simulink model "PMSM_PI_selfmode"  (R2023a)
settings: Solver=ode23tb  StartTime=0.0  StopTime=0.5  FixedStep=Ts  RelTol=1e-3  EnableMultiTasking=on
InitFcn:
  | Ts = 1e-6;
libraries: powerlib_extras x3, spsVoltageMeasurementLib x3, spsGroundLib x2, spsDCVoltageSourceLib x1, spsUniversalBridgeLib x1, simulink x1, spspowerguiLib x1
settings Model: Creator=Administrator  LastModifiedBy=Guoguo
settings SolverCC: AlgebraicLoopSolver=TrustRegion
settings DataIOCC: LimitDataPoints=on  SaveFormat=Array  SignalLoggingSaveFormat=ModelDataLogs  ReturnWorkspaceOutputs=off
settings OptimizationCC: ExpressionDepthLimit=2147483647  InitFltsAndDblsToZero=on  LifeSpan=inf
settings DebuggingCC: SaveWithParameterizedLinksMsg=none  UnderspecifiedInitializationDetection=Classic  MergeDetectMultiDrivingBlocksExec=none  SolverPrmCheckMsg=warning  FcnCallInpInsideContextMsg=warning  UnconnectedInputMsg=warning  UnconnectedOutputMsg=warning  UnconnectedLineMsg=warning  StateNameClashWarn=warning  SFUnexpectedBacktrackingDiag=warning  SFNoUnconditionalDefaultTransitionDiag=warning  SFExecutionAtInitializationDiag=none  ArithmeticOperatorsInVariantConditions=warning
settings HardwareCC: ProdBitPerPointer=32  ProdBitPerSizeT=32  ProdBitPerPtrDiffT=32  ProdLargestAtomicFloat=None  ProdIntDivRoundTo=Undefined  ProdEndianess=Unspecified  ProdWordSize=32  ProdHWDeviceType=32-bit Generic
settings ModelReferenceCC: EnableRefExpFcnMdlSchedulingChecks=on  PropagateSignalLabelsOutOfModel=off
settings SFSimCC: SimUseLocalCustomCode=off  CustomCodeUndefinedFunction=UseInterfaceOnly
settings RTWCC: RTWUseLocalCustomCode=off
settings CodeAppCC: StateflowObjectComments=on
settings GRTTargetCC: TargetFcnLib=ansi_tfl_tmw.mat  TargetLangStandard=C89/C90 (ANSI)  CombineOutputUpdateFcns=off  GRTInterface=on
settings ConfigComp: CovMetricSettings=dw  CovSaveCumulativeToWorkspaceVar=on  CovSaveSingleToWorkspaceVar=on  CovExternalEMLEnable=off  CovSFcnEnable=off
settings SimscapeCC: SimscapeNormalizeSystem=off

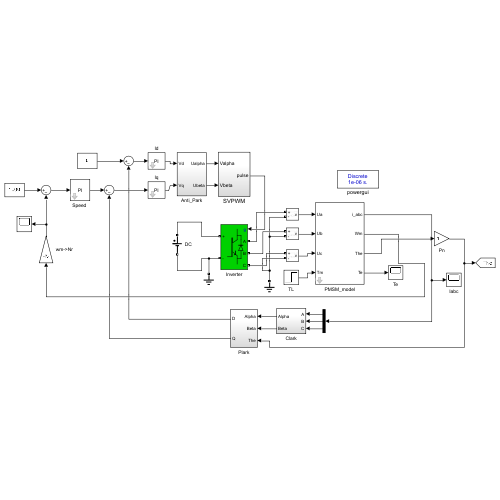
[thumbnail: Simulink's stored preview of the top-level diagram]
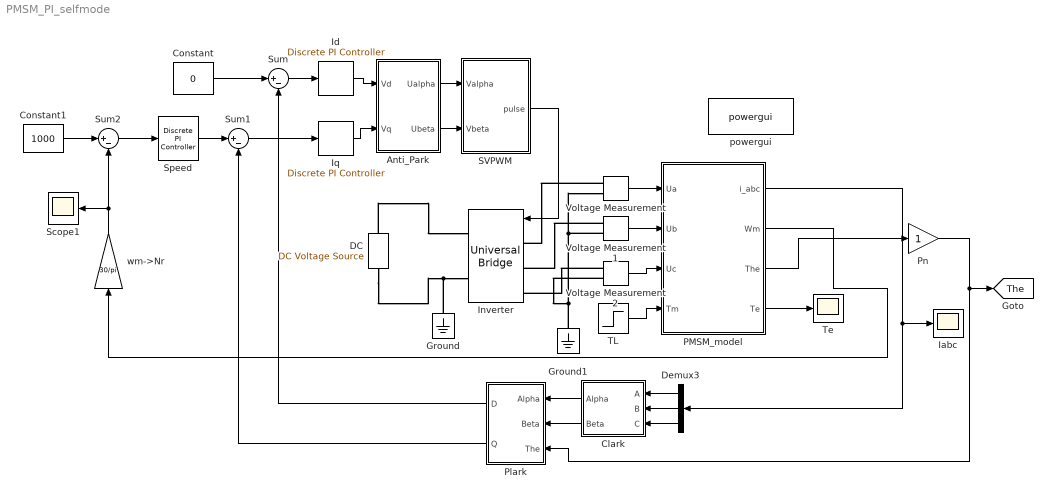
== system PMSM_PI_selfmode ==
  Anti_Park : Subsystem
  Clark : Subsystem
  Constant : Constant  Value=0
  Constant1 : Constant  Value=1000
  "DC " : spsDCVoltageSourceLib/DC Voltage Source  Amplitude=350  Measurements=None
  Demux3 : Demux  Outputs=3
  Ground : spsGroundLib/Ground  LConnTagsString=a
  Ground1 : spsGroundLib/Ground  LConnTagsString=a
  Iabc : Scope
  Id : powerlib_extras/Discrete  Control Blocks/Discrete PI Controller  Kp=8.8e-3*2200  Ki=2.875*2200  Par_Limits=[200 -200]  Init=0  Ts=Ts
  Inverter : spsUniversalBridgeLib/Universal Bridge  Arms=3  SnubberResistance=1e5  SnubberCapacitance=inf  Device=IGBT / Diodes  Ron=1e-3  Lon=0  ForwardVoltages="[  0  0  ]"  ForwardVoltage=0  GTOparameters=[ 10e-6 , 20e-6 ]  IGBTparameters=[ 1e-6 , 2e-6 ]  Measurements=None  Measurements_2=None  converterType=Rectifier
  Iq : powerlib_extras/Discrete  Control Blocks/Discrete PI Controller  Kp=8.5e-3*2200  Ki=2.875*20000  Par_Limits=[200 -200]  Init=0  Ts=Ts
  PMSM_model : Subsystem  mask{Ld=8.5e-3, Lq=8.5e-3, R=2.875, Pn=2, flux=0.533, B=0.0001, J=0.008}
      mask prompts: Ld "d-Inductances(Ld)"; Lq "q-Inductances(Lq)"; R "resistance(R)"; Pn "pole pairs(Pn)"; flux "Flux linkage(flux)"; B "viscous damping(B)"; J "Inertia(J)"
  Plark : Subsystem
  Pn : Gain
  SVPWM : Subsystem
  Scope1 : Scope
  "Speed " : powerlib_extras/Discrete  Control Blocks/Discrete PI Controller  Kp=0.2  Ki=10/4  Par_Limits=[15 -15]  Init=0  Ts=Ts
  Sum : Sum  Inputs=|+-
  Sum1 : Sum  Inputs=|+-
  Sum2 : Sum  Inputs=|+-
  TL : Step  Time=0.3  After=5  SampleTime=0
  Te : Scope
  Voltage Measurement : spsVoltageMeasurementLib/Voltage Measurement  PhasorSimulation=off  OutputType=Complex  PSBequivalent=0
  Voltage Measurement1 : spsVoltageMeasurementLib/Voltage Measurement  PhasorSimulation=off  OutputType=Complex  PSBequivalent=0
  Voltage Measurement2 : spsVoltageMeasurementLib/Voltage Measurement  PhasorSimulation=off  OutputType=Complex  PSBequivalent=0
  powergui : spspowerguiLib/powergui  SimulationMode=Discrete  SampleTime=Ts  frequency=60  Iterations=50  frequencyindice=0  Pbase=100e6  ErrMax=1e-4  UnitsV=kV  UnitsW=MW  buscounter=0  FunctionMessages=off  echomessages=off  EnableUseOfTLC=off  CurrentSourceSwitches=off  DisableSnubberDevices=off  DisableRonSwitches=off  DisableVfSwitches=off  DisplayEquations=off  AutomaticDiscreteSolvers=off  SolverType=Tustin/Backward Euler (TBE)  Interpol=off  ExternalGateDelay=off  methode=off  Ts=0  x0status=blocks  SPID=off  SwTol=0  HookPort=off  NonlinearTolerance=1e-4  nMaxIteration=100  ContinueOnMaxIteration=off  RestoreLinks=warning  ResistiveCurrentMeasurement=off  Frange=[0:2:500]  Ylog=off  Xlog=on  ShowGrid=off  save=off  variable=ZData  structure=0  ZoomFFT=off  StartTime=0.0  cycles=1  DisplayStyle=1  fundamental=60  FreqAxis=off  MaxFrequency=1000  frequencyindicesteady=1  RmsSteady=1  display=off
  wm->Nr : Gain  Gain=30/pi
  tag scope: The=global
  wires:
  SVPWM/1(pulse) -> Inverter/1
  Id/1 -> Anti_Park/1(Vd)
  Iq/1 -> Anti_Park/2(Vq)
  Sum/1 -> Id/1
  Sum1/1 -> Iq/1
  Sum2/1 -> "Speed "/1
  Constant1/1 -> Sum2/1
  "Speed "/1 -> Sum1/1
  wm->Nr/1 -> Sum2/2, Scope1/1
  Anti_Park/1(Ualpha) -> SVPWM/1(Valpha)
  Anti_Park/2(Ubeta) -> SVPWM/2(Vbeta)
  Constant/1 -> Sum/1
  Pn/1 -> Plark/3(The), [The]
  PMSM_model/3(The) -> Pn/1
  PMSM_model/2(Wm) -> wm->Nr/1
  PMSM_model/1(i_abc) -> Iabc/1, Demux3/1
  Clark/2(Beta) -> Plark/2(Beta)
  Clark/1(Alpha) -> Plark/1(Alpha)
  Demux3/1 -> Clark/1(A)
  Demux3/2 -> Clark/2(B)
  Demux3/3 -> Clark/3(C)
  Plark/1(D) -> Sum/2
  Plark/2(Q) -> Sum1/2
  Voltage Measurement/1 -> PMSM_model/1(Ua)
  Voltage Measurement1/1 -> PMSM_model/2(Ub)
  Voltage Measurement2/1 -> PMSM_model/3(Uc)
  TL/1 -> PMSM_model/4(Tm)
  PMSM_model/4(Te) -> Te/1
  connections:
  "DC "/RConn1 -- Inverter/RConn1
  "DC "/LConn1 -- Ground/LConn1 -- Inverter/RConn2
  Voltage Measurement/LConn1 -- Inverter/LConn1
  Voltage Measurement1/LConn1 -- Inverter/LConn2
  Voltage Measurement2/LConn1 -- Inverter/LConn3
  Ground1/LConn1 -- Voltage Measurement2/LConn2 -- Voltage Measurement1/LConn2 -- Voltage Measurement/LConn2

== system PMSM_PI_selfmode/Anti_Park ==
  Vd : Inport
  Vq : Inport  Port=2
  Fcn : Fcn  Expr=cos(u[1])*u[2]-sin(u[1])*u[3]
  Fcn1 : Fcn  Expr=sin(u[1])*u[2]+cos(u[1])*u[3]
  Mux1 : Mux  Inputs=3
  Ualpha : Outport  VectorParamsAs1DForOutWhenUnconnected=off
  Ubeta : Outport  Port=2  VectorParamsAs1DForOutWhenUnconnected=off
  wires:
  Fcn1/1 -> Ubeta/1
  Fcn/1 -> Ualpha/1
  Mux1/1 -> Fcn/1, Fcn1/1
  Vd/1 -> Mux1/2
  Vq/1 -> Mux1/3
  [The] -> Mux1/1

== system PMSM_PI_selfmode/Clark ==
  A : Inport
  B : Inport  Port=2
  C : Inport  Port=3
  Mux : Mux  Inputs=3
  alpha : Fcn  Expr=(u(1)-0.5*(u(2)+u(3)))*2/3
  beta : Fcn  Expr=sqrt(3)/2*(u(2)-u(3))*2/3
  Alpha : Outport  VectorParamsAs1DForOutWhenUnconnected=off
  Beta : Outport  Port=2  VectorParamsAs1DForOutWhenUnconnected=off
  wires:
  alpha/1 -> Alpha/1
  B/1 -> Mux/2
  C/1 -> Mux/3
  A/1 -> Mux/1
  Mux/1 -> beta/1, alpha/1
  beta/1 -> Beta/1

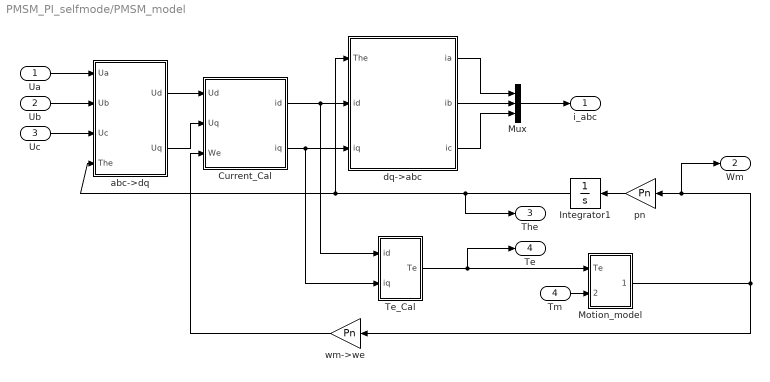
== system PMSM_PI_selfmode/PMSM_model ==
  Ua : Inport
  Ub : Inport  Port=2
  Uc : Inport  Port=3
  Tm : Inport  Port=4
  Current_Cal : Subsystem
  Integrator1 : Integrator
  Motion_model : Subsystem
  Mux : Mux  Inputs=3
  Te_Cal : Subsystem
  abc->dq : Subsystem
  dq->abc : Subsystem
  pn : Gain  Gain=Pn  SaturateOnIntegerOverflow=on  OutDataTypeStr=Inherit: Same as input  ParamDataTypeStr=Inherit: Same as input
  wm->we : Gain  Gain=Pn  SaturateOnIntegerOverflow=on  OutDataTypeStr=Inherit: Same as input  ParamDataTypeStr=Inherit: Same as input
  i_abc : Outport  VectorParamsAs1DForOutWhenUnconnected=off
  Wm : Outport  Port=2  VectorParamsAs1DForOutWhenUnconnected=off
  The : Outport  Port=3  VectorParamsAs1DForOutWhenUnconnected=off
  Te : Outport  Port=4  VectorParamsAs1DForOutWhenUnconnected=off
  wires:
  Ua/1 -> abc->dq/1(Ua)
  abc->dq/1(Ud) -> Current_Cal/1(Ud)
  abc->dq/2(Uq) -> Current_Cal/2(Uq)
  Current_Cal/1(id) -> Te_Cal/1(id), dq->abc/2(id)
  Current_Cal/2(iq) -> Te_Cal/2(iq), dq->abc/3(iq)
  Integrator1/1 -> abc->dq/4(The), dq->abc/1(The), The/1
  dq->abc/1(ia) -> Mux/1
  pn/1 -> Integrator1/1
  Uc/1 -> abc->dq/3(Uc)
  Ub/1 -> abc->dq/2(Ub)
  dq->abc/3(ic) -> Mux/3
  Mux/1 -> i_abc/1
  dq->abc/2(ib) -> Mux/2
  wm->we/1 -> Current_Cal/3(We)
  Motion_model/1(wm) -> wm->we/1, Wm/1, pn/1
  Te_Cal/1(Te) -> Te/1, Motion_model/1(Te)
  Tm/1 -> Motion_model/2(Tm)

== system PMSM_PI_selfmode/Plark ==
  Alpha : Inport
  Beta : Inport  Port=2
  The : Inport  Port=3
  Mux : Mux  Inputs=3
  d : Fcn  Expr=u(1)*cos(u(3))+u(2)*sin(u(3))
  q : Fcn  Expr=-u(1)*sin(u(3))+u(2)*cos(u(3))
  D : Outport  VectorParamsAs1DForOutWhenUnconnected=off
  Q : Outport  Port=2  VectorParamsAs1DForOutWhenUnconnected=off
  wires:
  d/1 -> D/1
  Beta/1 -> Mux/2
  The/1 -> Mux/3
  Alpha/1 -> Mux/1
  Mux/1 -> q/1, d/1
  q/1 -> Q/1

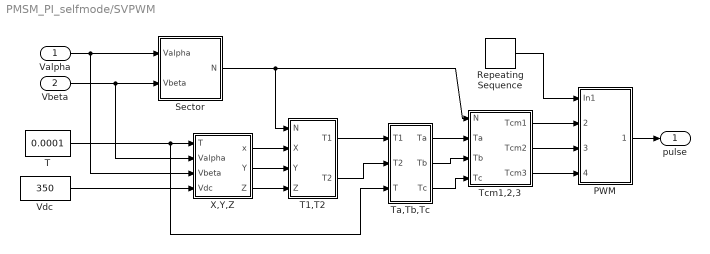
== system PMSM_PI_selfmode/SVPWM ==
  Valpha : Inport
  Vbeta : Inport  Port=2
  PWM : Subsystem
  Repeating Sequence : simulink/Sources/Repeating Sequence  rep_seq_t=[0 0.00005 0.0001]  rep_seq_y=[0 0.00005 0]
  Sector : Subsystem
  T : Constant  Value=0.0001
  T1,T2 : Subsystem
  Ta,Tb,Tc : Subsystem
  Tcm1,2,3 : Subsystem
  Vdc : Constant  Value=350
  X,Y,Z : Subsystem
  pulse : Outport  VectorParamsAs1DForOutWhenUnconnected=off
  wires:
  PWM/1(PWM) -> pulse/1
  Repeating Sequence/1 -> PWM/1(In1)
  Tcm1,2,3/3(Tcm3) -> PWM/4(Tcm3)
  Tcm1,2,3/2(Tcm2) -> PWM/3(Tcm2)
  Tcm1,2,3/1(Tcm1) -> PWM/2(Tcm1)
  Ta,Tb,Tc/3(Tc) -> Tcm1,2,3/4(Tc)
  Ta,Tb,Tc/2(Tb) -> Tcm1,2,3/3(Tb)
  Ta,Tb,Tc/1(Ta) -> Tcm1,2,3/2(Ta)
  T1,T2/2(T2) -> Ta,Tb,Tc/2(T2)
  T1,T2/1(T1) -> Ta,Tb,Tc/1(T1)
  X,Y,Z/3(Z) -> T1,T2/4(Z)
  X,Y,Z/2(Y) -> T1,T2/3(Y)
  X,Y,Z/1(x) -> T1,T2/2(X)
  Sector/1(N) -> T1,T2/1(N), Tcm1,2,3/1(N)
  Vdc/1 -> X,Y,Z/4(Vdc)
  T/1 -> Ta,Tb,Tc/3(T), X,Y,Z/1(T)
  Vbeta/1 -> X,Y,Z/2(Valpha), Sector/2(Vbeta)
  Valpha/1 -> X,Y,Z/3(Vbeta), Sector/1(Valpha)

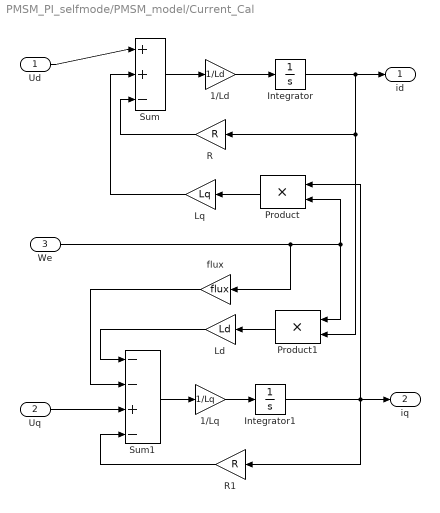
== system PMSM_PI_selfmode/PMSM_model/Current_Cal ==
  Ud : Inport
  Uq : Inport  Port=2
  We : Inport  Port=3
  1/Ld : Gain  Gain=1/Ld  SaturateOnIntegerOverflow=on  OutDataTypeStr=Inherit: Same as input  ParamDataTypeStr=Inherit: Same as input
  1/Lq : Gain  Gain=1/Lq  SaturateOnIntegerOverflow=on  OutDataTypeStr=Inherit: Same as input  ParamDataTypeStr=Inherit: Same as input
  Integrator : Integrator  InitialCondition=0.01
  Integrator1 : Integrator
  Ld : Gain  Gain=Ld  SaturateOnIntegerOverflow=on  OutDataTypeStr=Inherit: Same as input  ParamDataTypeStr=Inherit: Same as input
  Lq : Gain  Gain=Lq  SaturateOnIntegerOverflow=on  OutDataTypeStr=Inherit: Same as input  ParamDataTypeStr=Inherit: Same as input
  Product : Product  SaturateOnIntegerOverflow=on  OutDataTypeStr=Inherit: Same as first input
  Product1 : Product  SaturateOnIntegerOverflow=on  OutDataTypeStr=Inherit: Same as first input
  R : Gain  Gain=R  SaturateOnIntegerOverflow=on  OutDataTypeStr=Inherit: Same as input  ParamDataTypeStr=Inherit: Same as input
  R1 : Gain  Gain=R  SaturateOnIntegerOverflow=on  OutDataTypeStr=Inherit: Same as input  ParamDataTypeStr=Inherit: Same as input
  Sum : Sum  Inputs=|++-  SaturateOnIntegerOverflow=on
  Sum1 : Sum  Inputs=--+-  SaturateOnIntegerOverflow=on
  flux : Gain  Gain=flux  SaturateOnIntegerOverflow=on  OutDataTypeStr=Inherit: Same as input  ParamDataTypeStr=Inherit: Same as input
  id : Outport  VectorParamsAs1DForOutWhenUnconnected=off
  iq : Outport  Port=2  VectorParamsAs1DForOutWhenUnconnected=off
  wires:
  Ud/1 -> Sum/1
  Sum/1 -> 1/Ld/1
  1/Ld/1 -> Integrator/1
  Integrator/1 -> Product1/2, R/1, id/1
  Product/1 -> Lq/1
  Lq/1 -> Sum/2
  We/1 -> Product/2, Product1/1, flux/1
  R/1 -> Sum/3
  R1/1 -> Sum1/4
  1/Lq/1 -> Integrator1/1
  Sum1/1 -> 1/Lq/1
  Integrator1/1 -> R1/1, Product/1, iq/1
  Product1/1 -> Ld/1
  Ld/1 -> Sum1/1
  Uq/1 -> Sum1/3
  flux/1 -> Sum1/2

== system PMSM_PI_selfmode/PMSM_model/Motion_model ==
  Te : Inport
  Tm : Inport  Port=2
  1/J : Gain  Gain=1/J  SaturateOnIntegerOverflow=on  OutDataTypeStr=Inherit: Same as input  ParamDataTypeStr=Inherit: Same as input
  B : Gain  Gain=B  SaturateOnIntegerOverflow=on  OutDataTypeStr=Inherit: Same as input  ParamDataTypeStr=Inherit: Same as input
  Integrator : Integrator
  Memory : Memory
  Sum1 : Sum  Inputs=|+--  SaturateOnIntegerOverflow=on
  wm : Outport  VectorParamsAs1DForOutWhenUnconnected=off
  wires:
  Tm/1 -> Sum1/3
  Sum1/1 -> 1/J/1
  B/1 -> Sum1/2
  1/J/1 -> Integrator/1
  Te/1 -> Sum1/1
  Integrator/1 -> Memory/1, wm/1
  Memory/1 -> B/1

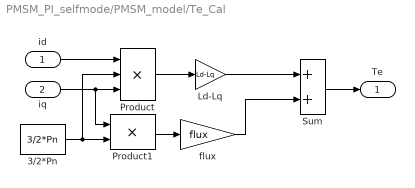
== system PMSM_PI_selfmode/PMSM_model/Te_Cal ==
  id : Inport
  iq : Inport  Port=2
  3/2*Pn : Constant  Value=3/2*Pn
  Ld-Lq : Gain  Gain=Ld-Lq  SaturateOnIntegerOverflow=on  OutDataTypeStr=Inherit: Same as input  ParamDataTypeStr=Inherit: Same as input
  Product : Product  Inputs=3  SaturateOnIntegerOverflow=on  OutDataTypeStr=Inherit: Same as first input
  Product1 : Product  SaturateOnIntegerOverflow=on  OutDataTypeStr=Inherit: Same as first input
  Sum : Sum  SaturateOnIntegerOverflow=on
  flux : Gain  Gain=flux  SaturateOnIntegerOverflow=on  OutDataTypeStr=Inherit: Same as input  ParamDataTypeStr=Inherit: Same as input
  Te : Outport  VectorParamsAs1DForOutWhenUnconnected=off
  wires:
  iq/1 -> Product1/1, Product/3
  id/1 -> Product/1
  Ld-Lq/1 -> Sum/1
  Product/1 -> Ld-Lq/1
  flux/1 -> Sum/2
  Product1/1 -> flux/1
  Sum/1 -> Te/1
  3/2*Pn/1 -> Product/2, Product1/2

== system PMSM_PI_selfmode/PMSM_model/abc->dq ==
  Ua : Inport
  Ub : Inport  Port=2
  Uc : Inport  Port=3
  The : Inport  Port=4
  Mux : Mux
  d : Fcn  Expr=(u(1)*cos(u(4))+u(2)*cos(u(4)-2/3*pi)+u(3)*cos(u(4)+2/3*pi))*2/3
  q : Fcn  Expr=-(u(1)*sin(u(4))+u(2)*sin(u(4)-2/3*pi)+u(3)*sin(u(4)+2/3*pi))*2/3
  Ud : Outport  VectorParamsAs1DForOutWhenUnconnected=off
  Uq : Outport  Port=2  VectorParamsAs1DForOutWhenUnconnected=off
  wires:
  Mux/1 -> q/1, d/1
  Ua/1 -> Mux/1
  Ub/1 -> Mux/2
  d/1 -> Ud/1
  The/1 -> Mux/4
  Uc/1 -> Mux/3
  q/1 -> Uq/1

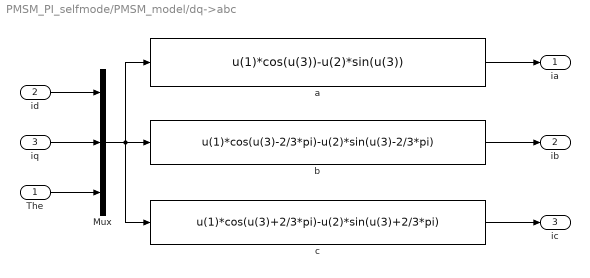
== system PMSM_PI_selfmode/PMSM_model/dq->abc ==
  The : Inport
  id : Inport  Port=2
  iq : Inport  Port=3
  Mux : Mux  Inputs=3
  a : Fcn  Expr=u(1)*cos(u(3))-u(2)*sin(u(3))
  b : Fcn  Expr=u(1)*cos(u(3)-2/3*pi)-u(2)*sin(u(3)-2/3*pi)
  c : Fcn  Expr=u(1)*cos(u(3)+2/3*pi)-u(2)*sin(u(3)+2/3*pi)
  ia : Outport  VectorParamsAs1DForOutWhenUnconnected=off
  ib : Outport  Port=2  VectorParamsAs1DForOutWhenUnconnected=off
  ic : Outport  Port=3  VectorParamsAs1DForOutWhenUnconnected=off
  wires:
  b/1 -> ib/1
  The/1 -> Mux/3
  a/1 -> ia/1
  id/1 -> Mux/1
  iq/1 -> Mux/2
  Mux/1 -> c/1, a/1, b/1
  c/1 -> ic/1

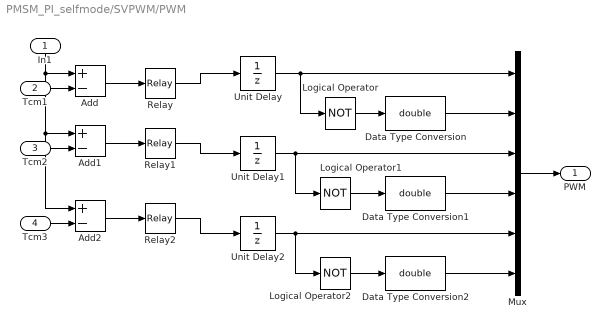
== system PMSM_PI_selfmode/SVPWM/PWM ==
  In1 : Inport
  Tcm1 : Inport  Port=2
  Tcm2 : Inport  Port=3
  Tcm3 : Inport  Port=4
  Add : Sum  Inputs=+-
  Add1 : Sum  Inputs=+-
  Add2 : Sum  Inputs=+-
  Data Type Conversion : DataTypeConversion  OutDataTypeStr=double  SaturateOnIntegerOverflow=off  RndMeth=Floor
  Data Type Conversion1 : DataTypeConversion  OutDataTypeStr=double  SaturateOnIntegerOverflow=off  RndMeth=Floor
  Data Type Conversion2 : DataTypeConversion  OutDataTypeStr=double  SaturateOnIntegerOverflow=off  RndMeth=Floor
  Logical Operator : Logic  Operator=NOT  AllPortsSameDT=off  OutDataTypeStr=boolean
  Logical Operator1 : Logic  Operator=NOT  AllPortsSameDT=off  OutDataTypeStr=boolean
  Logical Operator2 : Logic  Operator=NOT  AllPortsSameDT=off  OutDataTypeStr=boolean
  Mux : Mux  Inputs=6
  Relay : Relay  OffSwitchValue=-eps
  Relay1 : Relay  OffSwitchValue=-eps
  Relay2 : Relay  OffSwitchValue=-eps
  Unit Delay : UnitDelay  SampleTime=-1  HasFrameUpgradeWarning=on
  Unit Delay1 : UnitDelay  SampleTime=-1  HasFrameUpgradeWarning=on
  Unit Delay2 : UnitDelay  SampleTime=-1  HasFrameUpgradeWarning=on
  PWM : Outport  VectorParamsAs1DForOutWhenUnconnected=off
  wires:
  Tcm3/1 -> Add2/2
  Tcm2/1 -> Add1/2
  Tcm1/1 -> Add/2
  Relay2/1 -> Unit Delay2/1
  Relay1/1 -> Unit Delay1/1
  Relay/1 -> Unit Delay/1
  Unit Delay2/1 -> Mux/5, Logical Operator2/1
  Unit Delay1/1 -> Mux/3, Logical Operator1/1
  Unit Delay/1 -> Logical Operator/1, Mux/1
  Mux/1 -> PWM/1
  Data Type Conversion/1 -> Mux/2
  Data Type Conversion1/1 -> Mux/4
  Data Type Conversion2/1 -> Mux/6
  Logical Operator2/1 -> Data Type Conversion2/1
  Logical Operator1/1 -> Data Type Conversion1/1
  Logical Operator/1 -> Data Type Conversion/1
  Add1/1 -> Relay1/1
  Add2/1 -> Relay2/1
  Add/1 -> Relay/1
  In1/1 -> Add/1, Add2/1, Add1/1

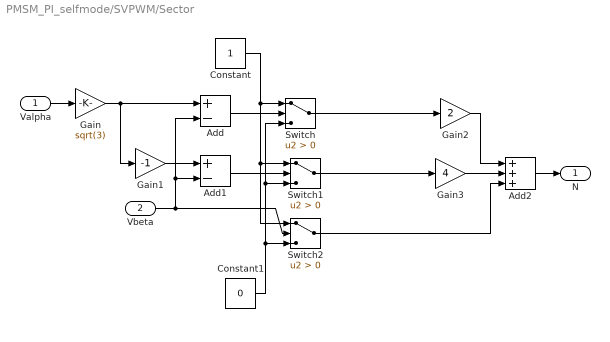
== system PMSM_PI_selfmode/SVPWM/Sector ==
  Valpha : Inport
  Vbeta : Inport  Port=2
  Add : Sum  Inputs=+-
  Add1 : Sum  Inputs=+-
  Add2 : Sum  Inputs=+++
  Constant : Constant
  Constant1 : Constant  Value=0
  Gain : Gain  Gain=sqrt(3)
  Gain1 : Gain  Gain=-1
  Gain2 : Gain  Gain=2
  Gain3 : Gain  Gain=4
  Switch : Switch  Criteria=u2 > Threshold  SaturateOnIntegerOverflow=off  InputSameDT=off
  Switch1 : Switch  Criteria=u2 > Threshold  SaturateOnIntegerOverflow=off  InputSameDT=off
  Switch2 : Switch  Criteria=u2 > Threshold  SaturateOnIntegerOverflow=off  InputSameDT=off
  N : Outport  VectorParamsAs1DForOutWhenUnconnected=off
  wires:
  Add2/1 -> N/1
  Valpha/1 -> Gain/1
  Gain3/1 -> Add2/2
  Gain2/1 -> Add2/1
  Add1/1 -> Switch1/2
  Gain1/1 -> Add1/1
  Switch1/1 -> Gain3/1
  Switch2/1 -> Add2/3
  Switch/1 -> Gain2/1
  Add/1 -> Switch/2
  Gain/1 -> Gain1/1, Add/1
  Constant1/1 -> Switch/3, Switch1/3, Switch2/3
  Constant/1 -> Switch1/1, Switch2/1, Switch/1
  Vbeta/1 -> Add1/2, Add/2, Switch2/2

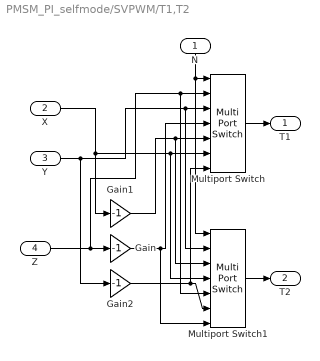
== system PMSM_PI_selfmode/SVPWM/T1,T2 ==
  N : Inport
  X : Inport  Port=2
  Y : Inport  Port=3
  Z : Inport  Port=4
  Gain : Gain  Gain=-1
  Gain1 : Gain  Gain=-1
  Gain2 : Gain  Gain=-1
  Multiport Switch : MultiPortSwitch  Inputs=6  SaturateOnIntegerOverflow=off  InputSameDT=off
  Multiport Switch1 : MultiPortSwitch  Inputs=6  SaturateOnIntegerOverflow=off  InputSameDT=off
  T1 : Outport  VectorParamsAs1DForOutWhenUnconnected=off
  T2 : Outport  Port=2  VectorParamsAs1DForOutWhenUnconnected=off
  wires:
  Multiport Switch1/1 -> T2/1
  Multiport Switch/1 -> T1/1
  Gain2/1 -> Multiport Switch/7, Multiport Switch1/6
  Gain1/1 -> Multiport Switch1/3, Multiport Switch/5
  X/1 -> Gain1/1, Multiport Switch/6, Multiport Switch1/4
  Gain/1 -> Multiport Switch1/7, Multiport Switch/4
  Y/1 -> Gain2/1, Multiport Switch1/2, Multiport Switch/3
  Z/1 -> Multiport Switch/2, Multiport Switch1/5, Gain/1
  N/1 -> Multiport Switch/1, Multiport Switch1/1

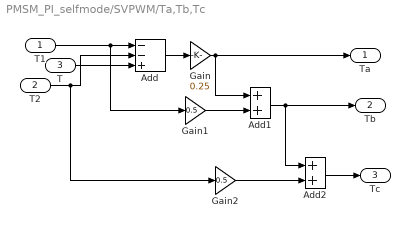
== system PMSM_PI_selfmode/SVPWM/Ta,Tb,Tc ==
  T1 : Inport
  T2 : Inport  Port=2
  T : Inport  Port=3
  Add : Sum  Inputs=--+
  Add1 : Sum
  Add2 : Sum
  Gain : Gain  Gain=0.25
  Gain1 : Gain  Gain=0.5
  Gain2 : Gain  Gain=0.5
  Ta : Outport  VectorParamsAs1DForOutWhenUnconnected=off
  Tb : Outport  Port=2  VectorParamsAs1DForOutWhenUnconnected=off
  Tc : Outport  Port=3  VectorParamsAs1DForOutWhenUnconnected=off
  wires:
  T/1 -> Add/3
  Add2/1 -> Tc/1
  Gain2/1 -> Add2/2
  Add1/1 -> Add2/1, Tb/1
  Gain1/1 -> Add1/2
  Gain/1 -> Add1/1, Ta/1
  Add/1 -> Gain/1
  T2/1 -> Add/2, Gain2/1
  T1/1 -> Add/1, Gain1/1

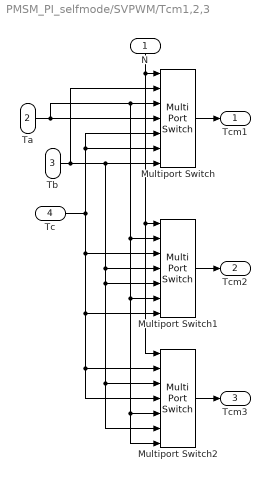
== system PMSM_PI_selfmode/SVPWM/Tcm1,2,3 ==
  N : Inport
  Ta : Inport  Port=2
  Tb : Inport  Port=3
  Tc : Inport  Port=4
  Multiport Switch : MultiPortSwitch  Inputs=6  SaturateOnIntegerOverflow=off  InputSameDT=off
  Multiport Switch1 : MultiPortSwitch  Inputs=6  SaturateOnIntegerOverflow=off  InputSameDT=off
  Multiport Switch2 : MultiPortSwitch  Inputs=6  SaturateOnIntegerOverflow=off  InputSameDT=off
  Tcm1 : Outport  VectorParamsAs1DForOutWhenUnconnected=off
  Tcm2 : Outport  Port=2  VectorParamsAs1DForOutWhenUnconnected=off
  Tcm3 : Outport  Port=3  VectorParamsAs1DForOutWhenUnconnected=off
  wires:
  Multiport Switch2/1 -> Tcm3/1
  Multiport Switch1/1 -> Tcm2/1
  Multiport Switch/1 -> Tcm1/1
  N/1 -> Multiport Switch2/1, Multiport Switch1/1, Multiport Switch/1
  Tc/1 -> Multiport Switch1/3, Multiport Switch1/7, Multiport Switch2/2, Multiport Switch2/4, Multiport Switch/5, Multiport Switch/6
  Ta/1 -> Multiport Switch/4, Multiport Switch/3, Multiport Switch1/2, Multiport Switch1/6, Multiport Switch2/5, Multiport Switch2/7
  Tb/1 -> Multiport Switch/2, Multiport Switch/7, Multiport Switch1/4, Multiport Switch1/5, Multiport Switch2/3, Multiport Switch2/6

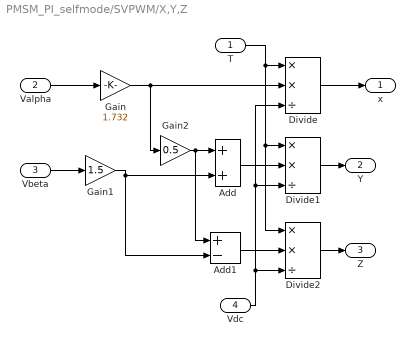
== system PMSM_PI_selfmode/SVPWM/X,Y,Z ==
  T : Inport
  Valpha : Inport  Port=2
  Vbeta : Inport  Port=3
  Vdc : Inport  Port=4
  Add : Sum
  Add1 : Sum  Inputs=+-
  Divide : Product  Inputs=**/
  Divide1 : Product  Inputs=**/
  Divide2 : Product  Inputs=**/
  Gain : Gain  Gain=1.732
  Gain1 : Gain  Gain=1.5
  Gain2 : Gain  Gain=0.5
  x : Outport  VectorParamsAs1DForOutWhenUnconnected=off
  Y : Outport  Port=2  VectorParamsAs1DForOutWhenUnconnected=off
  Z : Outport  Port=3  VectorParamsAs1DForOutWhenUnconnected=off
  wires:
  Divide2/1 -> Z/1
  Divide1/1 -> Y/1
  Divide/1 -> x/1
  Vbeta/1 -> Gain1/1
  Valpha/1 -> Gain/1
  Add1/1 -> Divide2/2
  Add/1 -> Divide1/2
  Gain1/1 -> Add1/2, Add/2
  Gain2/1 -> Add1/1, Add/1
  Gain/1 -> Gain2/1, Divide/2
  Vdc/1 -> Divide/3, Divide1/3, Divide2/3
  T/1 -> Divide2/1, Divide1/1, Divide/1
